simulink model "solar"  (R2018a)
settings: Solver=VariableStepDiscrete  StartTime=0.0  StopTime=1  RelTol=1e-3
undefined symbols (not defined in the file): G, Insolation, Io, Ns, Rp, Rs
libraries: simulink x10, powerlib x1
settings Model: Creator=zxyxi  LastModifiedBy=zxyxi

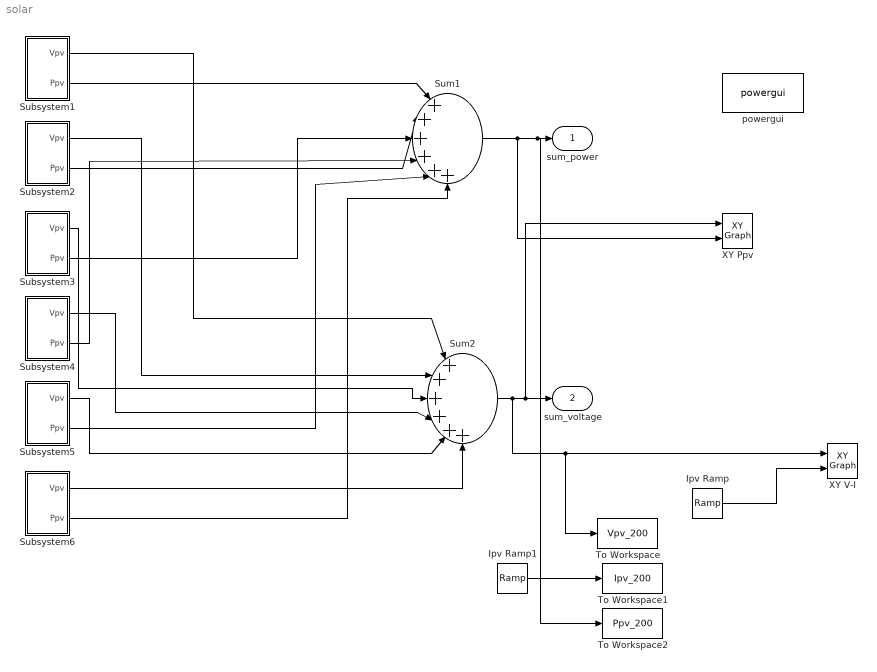
== system solar ==
  Ipv Ramp : simulink/Sources/Ramp  slope=6  start=0  InitialOutput=0
  Ipv Ramp1 : simulink/Sources/Ramp  slope=6  start=0  InitialOutput=0
  Subsystem1 : Subsystem
  Subsystem2 : Subsystem
  Subsystem3 : Subsystem
  Subsystem4 : Subsystem
  Subsystem5 : Subsystem
  Subsystem6 : Subsystem
  Sum1 : Sum  Inputs=|++++++
  Sum2 : Sum  Inputs=|++++++
  To Workspace : ToWorkspace  VariableName=Vpv_200  SaveFormat=Timeseries  SampleTime=-1
  To Workspace1 : ToWorkspace  VariableName=Ipv_200  SaveFormat=Timeseries  SampleTime=-1
  To Workspace2 : ToWorkspace  VariableName=Ppv_200  SaveFormat=Timeseries  SampleTime=-1
  XY Ppv : simulink/Sinks/XY Graph  xmin=0  xmax=150  ymin=0  ymax=500  st=-1
  XY V-I : simulink/Sinks/XY Graph  xmin=0  xmax=150  ymin=0  ymax=6  st=-1
  powergui : powerlib/powergui  Priority=1  SimulationMode=Continuous  SampleTime=50e-10  frequency=60  Iterations=50  frequencyindice=60  Pbase=100e6  ErrMax=1e-4  UnitsV=kV  UnitsW=MW  buscounter=0  FunctionMessages=off  echomessages=off  EnableUseOfTLC=off  CurrentSourceSwitches=off  DisableSnubberDevices=off  DisableRonSwitches=off  DisableVfSwitches=off  DisplayEquations=off  SolverType=Tustin/Backward Euler (TBE)  Interpol=off  ExternalGateDelay=off  methode=off  Ts=100  x0status=blocks  SPID=on  SwTol=0  HookPort=off  RestoreLinks=warning  ResistiveCurrentMeasurement=off  Frange=[0:2:500]  Ylog=off  Xlog=on  ShowGrid=off  save=off  variable=ZData  structure=0  ZoomFFT=off  StartTime=0.0  cycles=1  DisplayStyle=1  fundamental=60  FreqAxis=off  MaxFrequency=1000  frequencyindicesteady=1  RmsSteady=1  display=off
  "sum_power " : Outport
  "sum_voltage " : Outport  Port=2
  wires:
  Subsystem1/2(Ppv) -> Sum1/1
  Subsystem2/2(Ppv) -> Sum1/2
  Subsystem3/2(Ppv) -> Sum1/3
  Subsystem4/2(Ppv) -> Sum1/4
  Subsystem5/2(Ppv) -> Sum1/5
  Subsystem6/2(Ppv) -> Sum1/6
  Subsystem1/1(Vpv) -> Sum2/1
  Subsystem2/1(Vpv) -> Sum2/2
  Subsystem3/1(Vpv) -> Sum2/3
  Subsystem4/1(Vpv) -> Sum2/4
  Subsystem5/1(Vpv) -> Sum2/5
  Subsystem6/1(Vpv) -> Sum2/6
  Sum1/1 -> To Workspace2/1, "sum_power "/1, XY Ppv/2
  Sum2/1 -> To Workspace/1, XY V-I/1, XY Ppv/1, "sum_voltage "/1
  Ipv Ramp/1 -> XY V-I/2
  Ipv Ramp1/1 -> To Workspace1/1

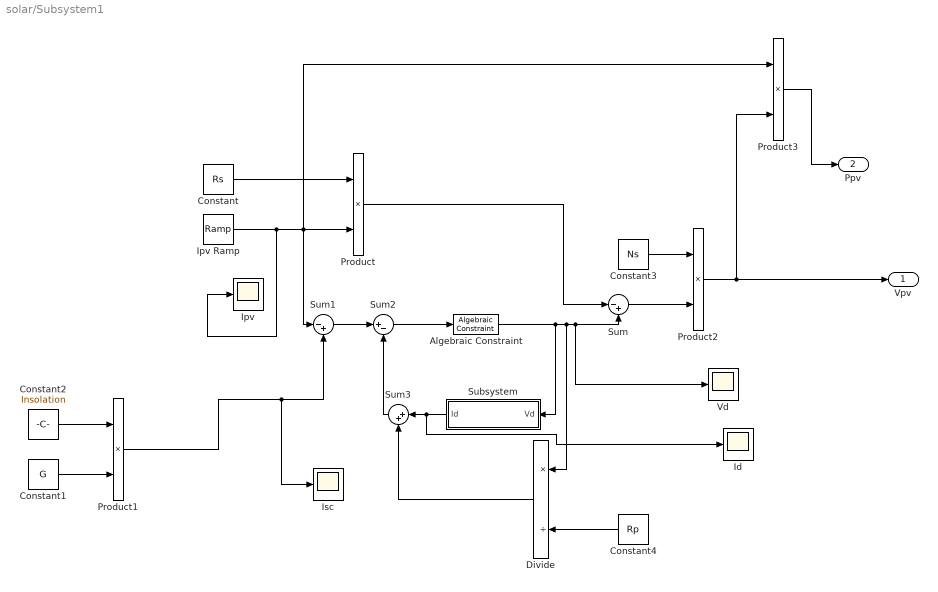
== system solar/Subsystem1 ==
  Algebraic Constraint : AlgebraicConstraint
  Constant : Constant  Value=Rs
  Constant1 : Constant  Value=G
  Constant2 : Constant  Value=Insolation
  Constant3 : Constant  Value=Ns
  Constant4 : Constant  Value=Rp
  Divide : Product  Inputs=*/
  Id : Scope
  "Ipv " : Scope
  Ipv Ramp : simulink/Sources/Ramp  slope=6  start=0  InitialOutput=0
  Isc : Scope
  Product{,1..3} (4 alike) : Product
  Subsystem : Subsystem
  Sum : Sum  Inputs=|-+
  Sum1 : Sum  Inputs=|-+
  Sum2 : Sum  Inputs=|+-
  Sum3 : Sum  Inputs=|++
  Vd : Scope
  Vpv : Outport
  Ppv : Outport  Port=2
  wires:
  Sum2/1 -> Algebraic Constraint/1
  Sum/1 -> Product2/2
  Subsystem/1(Id) -> Id/1, Sum3/1
  Constant4/1 -> Divide/2
  Product1/1 -> Isc/1, Sum1/2
  Constant1/1 -> Product1/2
  Product2/1 -> Vpv/1, Product3/2
  Product3/1 -> Ppv/1
  Sum1/1 -> Sum2/1
  Ipv Ramp/1 -> "Ipv "/1, Product3/1, Sum1/1, Product/2
  Constant2/1 -> Product1/1
  Algebraic Constraint/1 -> Subsystem/1(Vd), Divide/1, Vd/1, Sum/2
  Constant/1 -> Product/1
  Product/1 -> Sum/1
  Constant3/1 -> Product2/1
  Sum3/1 -> Sum2/2
  Divide/1 -> Sum3/2

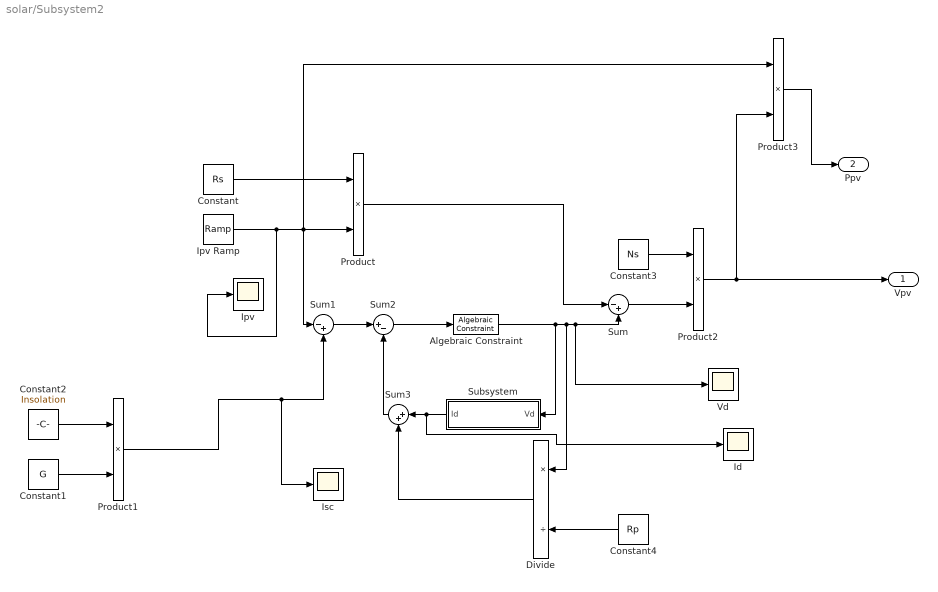
== system solar/Subsystem2 ==
  Algebraic Constraint : AlgebraicConstraint
  Constant : Constant  Value=Rs
  Constant1 : Constant  Value=G
  Constant2 : Constant  Value=Insolation
  Constant3 : Constant  Value=Ns
  Constant4 : Constant  Value=Rp
  Divide : Product  Inputs=*/
  Id : Scope
  "Ipv " : Scope
  Ipv Ramp : simulink/Sources/Ramp  slope=6  start=0  InitialOutput=0
  Isc : Scope
  Product{,1..3} (4 alike) : Product
  Subsystem : Subsystem
  Sum : Sum  Inputs=|-+
  Sum1 : Sum  Inputs=|-+
  Sum2 : Sum  Inputs=|+-
  Sum3 : Sum  Inputs=|++
  Vd : Scope
  Vpv : Outport
  Ppv : Outport  Port=2
  wires:
  Sum2/1 -> Algebraic Constraint/1
  Sum/1 -> Product2/2
  Subsystem/1(Id) -> Id/1, Sum3/1
  Constant4/1 -> Divide/2
  Product1/1 -> Isc/1, Sum1/2
  Constant1/1 -> Product1/2
  Product2/1 -> Vpv/1, Product3/2
  Product3/1 -> Ppv/1
  Sum1/1 -> Sum2/1
  Ipv Ramp/1 -> "Ipv "/1, Product3/1, Sum1/1, Product/2
  Constant2/1 -> Product1/1
  Algebraic Constraint/1 -> Subsystem/1(Vd), Divide/1, Vd/1, Sum/2
  Constant/1 -> Product/1
  Product/1 -> Sum/1
  Constant3/1 -> Product2/1
  Sum3/1 -> Sum2/2
  Divide/1 -> Sum3/2

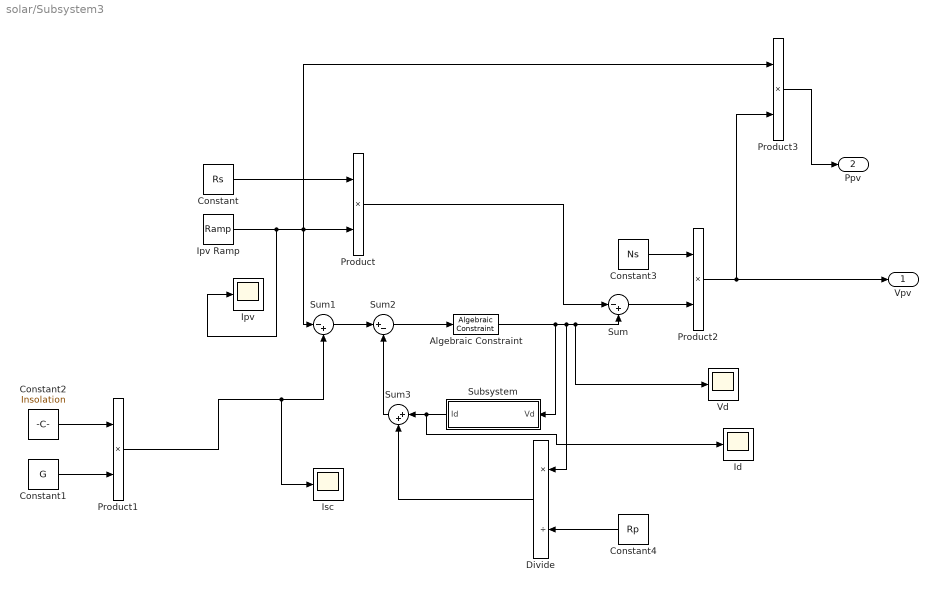
== system solar/Subsystem3 ==
  Algebraic Constraint : AlgebraicConstraint
  Constant : Constant  Value=Rs
  Constant1 : Constant  Value=G
  Constant2 : Constant  Value=Insolation
  Constant3 : Constant  Value=Ns
  Constant4 : Constant  Value=Rp
  Divide : Product  Inputs=*/
  Id : Scope
  "Ipv " : Scope
  Ipv Ramp : simulink/Sources/Ramp  slope=6  start=0  InitialOutput=0
  Isc : Scope
  Product{,1..3} (4 alike) : Product
  Subsystem : Subsystem
  Sum : Sum  Inputs=|-+
  Sum1 : Sum  Inputs=|-+
  Sum2 : Sum  Inputs=|+-
  Sum3 : Sum  Inputs=|++
  Vd : Scope
  Vpv : Outport
  Ppv : Outport  Port=2
  wires:
  Sum2/1 -> Algebraic Constraint/1
  Sum/1 -> Product2/2
  Subsystem/1(Id) -> Id/1, Sum3/1
  Constant4/1 -> Divide/2
  Product1/1 -> Isc/1, Sum1/2
  Constant1/1 -> Product1/2
  Product2/1 -> Vpv/1, Product3/2
  Product3/1 -> Ppv/1
  Sum1/1 -> Sum2/1
  Ipv Ramp/1 -> "Ipv "/1, Product3/1, Sum1/1, Product/2
  Constant2/1 -> Product1/1
  Algebraic Constraint/1 -> Subsystem/1(Vd), Divide/1, Vd/1, Sum/2
  Constant/1 -> Product/1
  Product/1 -> Sum/1
  Constant3/1 -> Product2/1
  Sum3/1 -> Sum2/2
  Divide/1 -> Sum3/2

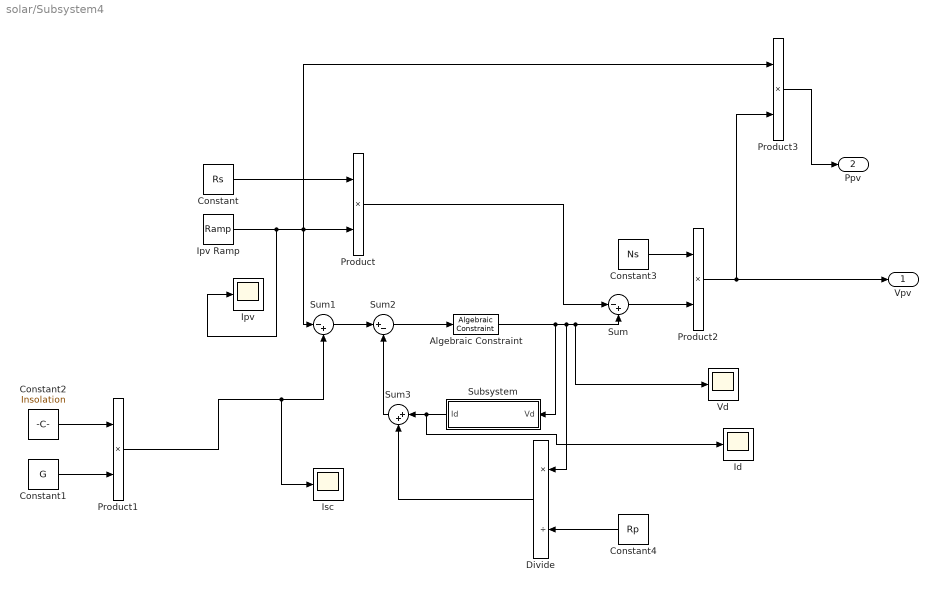
== system solar/Subsystem4 ==
  Algebraic Constraint : AlgebraicConstraint
  Constant : Constant  Value=Rs
  Constant1 : Constant  Value=G
  Constant2 : Constant  Value=Insolation
  Constant3 : Constant  Value=Ns
  Constant4 : Constant  Value=Rp
  Divide : Product  Inputs=*/
  Id : Scope
  "Ipv " : Scope
  Ipv Ramp : simulink/Sources/Ramp  slope=6  start=0  InitialOutput=0
  Isc : Scope
  Product{,1..3} (4 alike) : Product
  Subsystem : Subsystem
  Sum : Sum  Inputs=|-+
  Sum1 : Sum  Inputs=|-+
  Sum2 : Sum  Inputs=|+-
  Sum3 : Sum  Inputs=|++
  Vd : Scope
  Vpv : Outport
  Ppv : Outport  Port=2
  wires:
  Sum2/1 -> Algebraic Constraint/1
  Sum/1 -> Product2/2
  Subsystem/1(Id) -> Id/1, Sum3/1
  Constant4/1 -> Divide/2
  Product1/1 -> Isc/1, Sum1/2
  Constant1/1 -> Product1/2
  Product2/1 -> Vpv/1, Product3/2
  Product3/1 -> Ppv/1
  Sum1/1 -> Sum2/1
  Ipv Ramp/1 -> "Ipv "/1, Product3/1, Sum1/1, Product/2
  Constant2/1 -> Product1/1
  Algebraic Constraint/1 -> Subsystem/1(Vd), Divide/1, Vd/1, Sum/2
  Constant/1 -> Product/1
  Product/1 -> Sum/1
  Constant3/1 -> Product2/1
  Sum3/1 -> Sum2/2
  Divide/1 -> Sum3/2

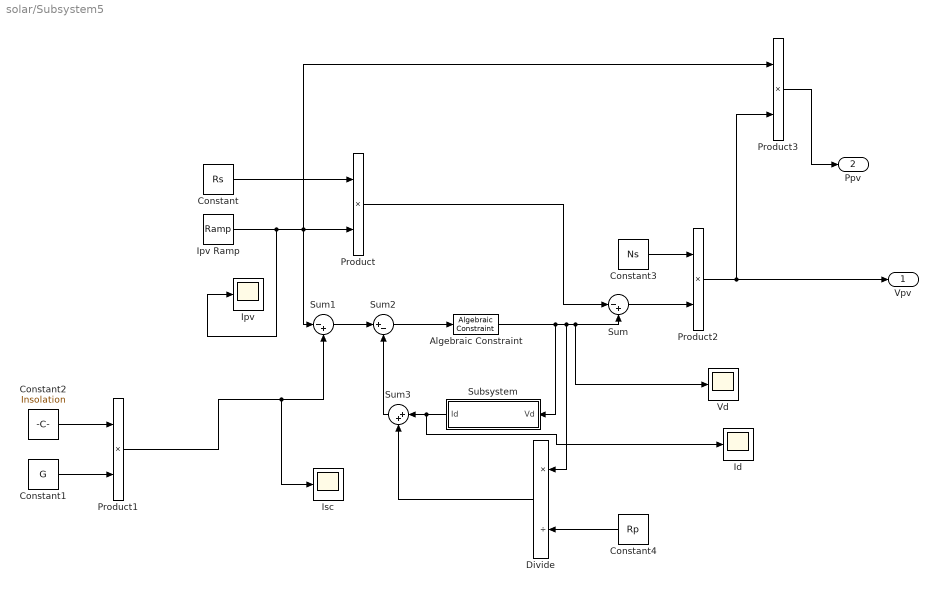
== system solar/Subsystem5 ==
  Algebraic Constraint : AlgebraicConstraint
  Constant : Constant  Value=Rs
  Constant1 : Constant  Value=G
  Constant2 : Constant  Value=Insolation
  Constant3 : Constant  Value=Ns
  Constant4 : Constant  Value=Rp
  Divide : Product  Inputs=*/
  Id : Scope
  "Ipv " : Scope
  Ipv Ramp : simulink/Sources/Ramp  slope=6  start=0  InitialOutput=0
  Isc : Scope
  Product{,1..3} (4 alike) : Product
  Subsystem : Subsystem
  Sum : Sum  Inputs=|-+
  Sum1 : Sum  Inputs=|-+
  Sum2 : Sum  Inputs=|+-
  Sum3 : Sum  Inputs=|++
  Vd : Scope
  Vpv : Outport
  Ppv : Outport  Port=2
  wires:
  Sum2/1 -> Algebraic Constraint/1
  Sum/1 -> Product2/2
  Subsystem/1(Id) -> Id/1, Sum3/1
  Constant4/1 -> Divide/2
  Product1/1 -> Isc/1, Sum1/2
  Constant1/1 -> Product1/2
  Product2/1 -> Vpv/1, Product3/2
  Product3/1 -> Ppv/1
  Sum1/1 -> Sum2/1
  Ipv Ramp/1 -> "Ipv "/1, Product3/1, Sum1/1, Product/2
  Constant2/1 -> Product1/1
  Algebraic Constraint/1 -> Subsystem/1(Vd), Divide/1, Vd/1, Sum/2
  Constant/1 -> Product/1
  Product/1 -> Sum/1
  Constant3/1 -> Product2/1
  Sum3/1 -> Sum2/2
  Divide/1 -> Sum3/2

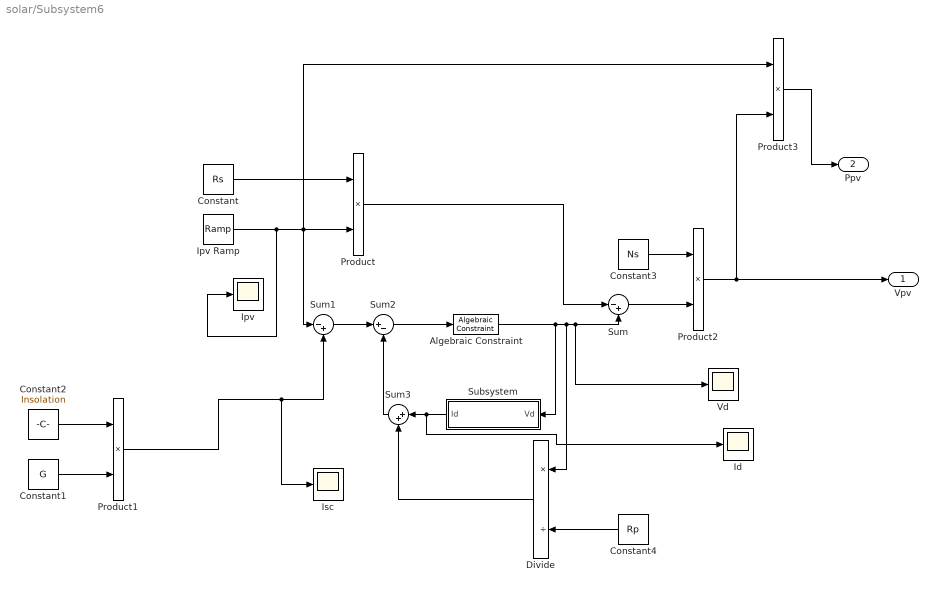
== system solar/Subsystem6 ==
  Algebraic Constraint : AlgebraicConstraint
  Constant : Constant  Value=Rs
  Constant1 : Constant  Value=G
  Constant2 : Constant  Value=Insolation
  Constant3 : Constant  Value=Ns
  Constant4 : Constant  Value=Rp
  Divide : Product  Inputs=*/
  Id : Scope
  "Ipv " : Scope
  Ipv Ramp : simulink/Sources/Ramp  slope=6  start=0  InitialOutput=0
  Isc : Scope
  Product{,1..3} (4 alike) : Product
  Subsystem : Subsystem
  Sum : Sum  Inputs=|-+
  Sum1 : Sum  Inputs=|-+
  Sum2 : Sum  Inputs=|+-
  Sum3 : Sum  Inputs=|++
  Vd : Scope
  Vpv : Outport
  Ppv : Outport  Port=2
  wires:
  Sum2/1 -> Algebraic Constraint/1
  Sum/1 -> Product2/2
  Subsystem/1(Id) -> Id/1, Sum3/1
  Constant4/1 -> Divide/2
  Product1/1 -> Isc/1, Sum1/2
  Constant1/1 -> Product1/2
  Product2/1 -> Vpv/1, Product3/2
  Product3/1 -> Ppv/1
  Sum1/1 -> Sum2/1
  Ipv Ramp/1 -> "Ipv "/1, Product3/1, Sum1/1, Product/2
  Constant2/1 -> Product1/1
  Algebraic Constraint/1 -> Subsystem/1(Vd), Divide/1, Vd/1, Sum/2
  Constant/1 -> Product/1
  Product/1 -> Sum/1
  Constant3/1 -> Product2/1
  Sum3/1 -> Sum2/2
  Divide/1 -> Sum3/2

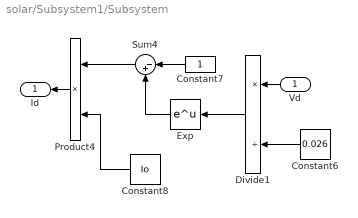
== system solar/Subsystem1/Subsystem ==
  Vd : Inport
  Constant6 : Constant  Value=0.026
  Constant7 : Constant
  Constant8 : Constant  Value=Io
  Divide1 : Product  Inputs=*/
  Exp : Math  SaturateOnIntegerOverflow=on
  Product4 : Product
  Sum4 : Sum  Inputs=|-+
  Id : Outport
  wires:
  Constant7/1 -> Sum4/1
  Vd/1 -> Divide1/1
  Constant6/1 -> Divide1/2
  Product4/1 -> Id/1
  Sum4/1 -> Product4/1
  Constant8/1 -> Product4/2
  Divide1/1 -> Exp/1
  Exp/1 -> Sum4/2

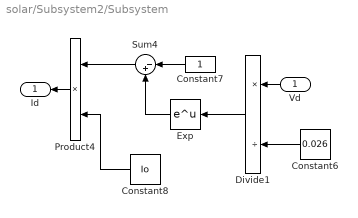
== system solar/Subsystem2/Subsystem ==
  Vd : Inport
  Constant6 : Constant  Value=0.026
  Constant7 : Constant
  Constant8 : Constant  Value=Io
  Divide1 : Product  Inputs=*/
  Exp : Math  SaturateOnIntegerOverflow=on
  Product4 : Product
  Sum4 : Sum  Inputs=|-+
  Id : Outport
  wires:
  Constant7/1 -> Sum4/1
  Vd/1 -> Divide1/1
  Constant6/1 -> Divide1/2
  Product4/1 -> Id/1
  Sum4/1 -> Product4/1
  Constant8/1 -> Product4/2
  Divide1/1 -> Exp/1
  Exp/1 -> Sum4/2

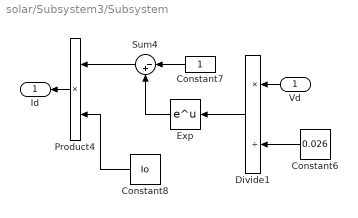
== system solar/Subsystem3/Subsystem ==
  Vd : Inport
  Constant6 : Constant  Value=0.026
  Constant7 : Constant
  Constant8 : Constant  Value=Io
  Divide1 : Product  Inputs=*/
  Exp : Math  SaturateOnIntegerOverflow=on
  Product4 : Product
  Sum4 : Sum  Inputs=|-+
  Id : Outport
  wires:
  Constant7/1 -> Sum4/1
  Vd/1 -> Divide1/1
  Constant6/1 -> Divide1/2
  Product4/1 -> Id/1
  Sum4/1 -> Product4/1
  Constant8/1 -> Product4/2
  Divide1/1 -> Exp/1
  Exp/1 -> Sum4/2

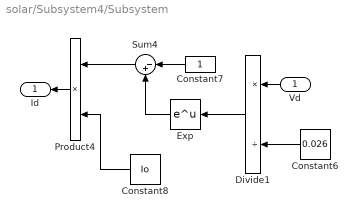
== system solar/Subsystem4/Subsystem ==
  Vd : Inport
  Constant6 : Constant  Value=0.026
  Constant7 : Constant
  Constant8 : Constant  Value=Io
  Divide1 : Product  Inputs=*/
  Exp : Math  SaturateOnIntegerOverflow=on
  Product4 : Product
  Sum4 : Sum  Inputs=|-+
  Id : Outport
  wires:
  Constant7/1 -> Sum4/1
  Vd/1 -> Divide1/1
  Constant6/1 -> Divide1/2
  Product4/1 -> Id/1
  Sum4/1 -> Product4/1
  Constant8/1 -> Product4/2
  Divide1/1 -> Exp/1
  Exp/1 -> Sum4/2

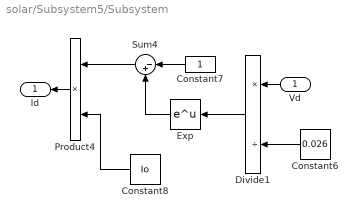
== system solar/Subsystem5/Subsystem ==
  Vd : Inport
  Constant6 : Constant  Value=0.026
  Constant7 : Constant
  Constant8 : Constant  Value=Io
  Divide1 : Product  Inputs=*/
  Exp : Math  SaturateOnIntegerOverflow=on
  Product4 : Product
  Sum4 : Sum  Inputs=|-+
  Id : Outport
  wires:
  Constant7/1 -> Sum4/1
  Vd/1 -> Divide1/1
  Constant6/1 -> Divide1/2
  Product4/1 -> Id/1
  Sum4/1 -> Product4/1
  Constant8/1 -> Product4/2
  Divide1/1 -> Exp/1
  Exp/1 -> Sum4/2

== system solar/Subsystem6/Subsystem ==
  Vd : Inport
  Constant6 : Constant  Value=0.026
  Constant7 : Constant
  Constant8 : Constant  Value=Io
  Divide1 : Product  Inputs=*/
  Exp : Math  SaturateOnIntegerOverflow=on
  Product4 : Product
  Sum4 : Sum  Inputs=|-+
  Id : Outport
  wires:
  Constant7/1 -> Sum4/1
  Vd/1 -> Divide1/1
  Constant6/1 -> Divide1/2
  Product4/1 -> Id/1
  Sum4/1 -> Product4/1
  Constant8/1 -> Product4/2
  Divide1/1 -> Exp/1
  Exp/1 -> Sum4/2
